simulink library "ob_alb_fov"  (Simulink 6.2)
undefined symbols (not defined in the file or in its folder): albedo_onboard_wrapper, zenith2ref
libraries: components_lib x5, simulink x1, sensor_emulation_lib x1
settings Model: Creator=rsni02  LastModifiedBy=rsni02  ExtModeAutoUpdateStatusClock=off

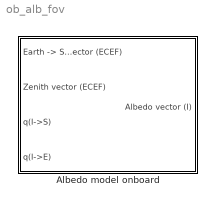
== system ob_alb_fov ==
  Albedo model onboard : Subsystem  mask{sun_flux=1366.9, matrix=FOV cosine dep. reflectivity table, enable=off}
      mask prompts: sun_flux "Sun flux (mean: 1366.9)"; matrix "Choose used reflectivity data:"; enable "Use reflectivity matrix (blackbox)"
      mask init:
      | if matrix == 1
      |     mrm = load('fov_albedo_matrix.mat');
      |     mrm = mrm.mrm;  
      | elseif matrix == 2
      |     mrm = load('fov_meaned_albedo_matrix.mat');
      |     mrm = mrm.mrm;
      | elseif matrix == 3
      |     mrm = load('fov_albedo_polynomial_matrix.mat');
      |     mrm = mrm.mrm;
      | elseif matrix == 4
      |     mrm = ones(180,288).*0.30;
      | end
      mask StyleString: edit,popup(FOV cosine dep. reflectivity table|FOV meaned reflectivity table|Polynomial fit to latitude meaned reflectivity|Constant reflectivity of 30%),checkbox

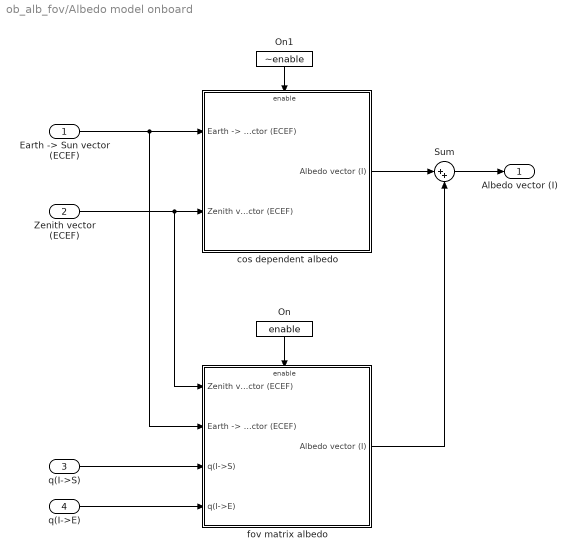
== system ob_alb_fov/Albedo model onboard ==
  "Earth -> Sun vector (ECEF)" : Inport  Port=1  LatchInput=off
  Zenith vector (ECEF) : Inport  Port=2  LatchInput=off
  q(I->S) : Inport  Port=3  LatchInput=off
  q(I->E) : Inport  Port=4  LatchInput=off
  On : Constant  Orientation=down  Value=enable
  On1 : Constant  Orientation=down  Value=~enable
  Sum : Sum  Inputs=|++
  cos dependent albedo : Subsystem
  fov matrix albedo : Subsystem
  Albedo vector (I) : Outport
  wires:
  On1/1 -> cos dependent albedo/Enable
  fov matrix albedo/1(Albedo vector (I)) -> Sum/2
  cos dependent albedo/1(Albedo vector (I)) -> Sum/1
  On/1 -> fov matrix albedo/Enable
  Zenith vector (ECEF)/1 -> fov matrix albedo/1(Zenith vector (ECEF)), cos dependent albedo/2(Zenith vector (ECEF))
  "Earth -> Sun vector (ECEF)"/1 -> fov matrix albedo/2("Earth -> Sun vector (ECEF)"), cos dependent albedo/1("Earth -> Sun vector (ECEF)")
  q(I->E)/1 -> fov matrix albedo/4(q(I->E))
  q(I->S)/1 -> fov matrix albedo/3(q(I->S))
  Sum/1 -> Albedo vector (I)/1

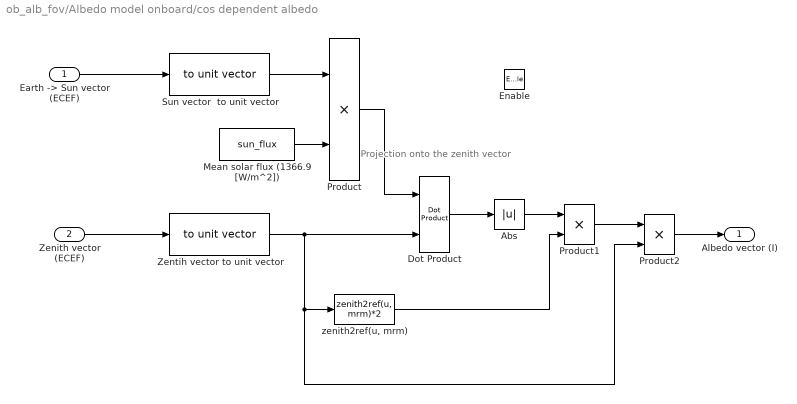
== system ob_alb_fov/Albedo model onboard/cos dependent albedo ==
  note: Projection onto
      | the zenith vector
  "Earth -> Sun vector (ECEF)" : Inport  Port=1  LatchInput=off
  Zenith vector (ECEF) : Inport  Port=2  LatchInput=off
  Enable : EnablePort  StatesWhenEnabling=reset
  Abs : Abs
  Dot Product : simulink/Math Operations/Dot Product  InputSameDT=on  OutDataType=sfix(16)  OutScaling=2^-10  DoSatur=off
  Mean solar flux (1366.9 [W/m^2]) : Constant  Value=sun_flux
  Product : Product  RndMeth=Zero
  Product1 : Product  RndMeth=Zero
  Product2 : Product  RndMeth=Zero
  Sun vector  to unit vector : components_lib/Math utilities/Vector operations/to unit vector
  Zentih vector to unit vector : components_lib/Math utilities/Vector operations/to unit vector
  "zenith2ref(u, mrm)" : MATLABFcn  MATLABFcn=zenith2ref(u, mrm)*2
  Albedo vector (I) : Outport
  wires:
  Product2/1 -> Albedo vector (I)/1
  Product1/1 -> Product2/1
  Abs/1 -> Product1/1
  Dot Product/1 -> Abs/1
  Sun vector  to unit vector/1 -> Product/1
  Mean solar flux (1366.9 [W/m^2])/1 -> Product/2
  Product/1 -> Dot Product/1
  "zenith2ref(u, mrm)"/1 -> Product1/2
  Zentih vector to unit vector/1 -> Product2/2, "zenith2ref(u, mrm)"/1, Dot Product/2
  "Earth -> Sun vector (ECEF)"/1 -> Sun vector  to unit vector/1
  Zenith vector (ECEF)/1 -> Zentih vector to unit vector/1

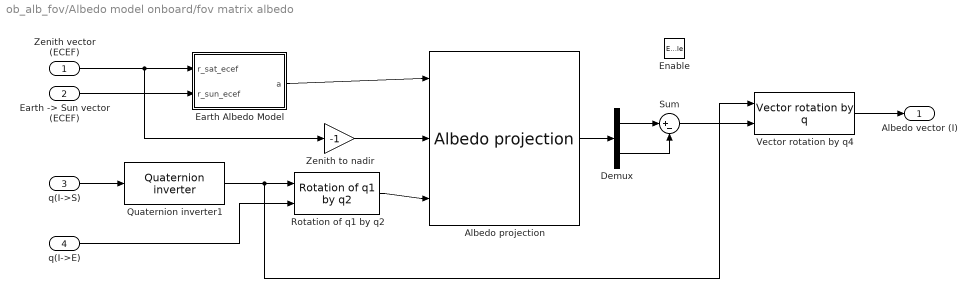
== system ob_alb_fov/Albedo model onboard/fov matrix albedo ==
  Zenith vector (ECEF) : Inport  Port=1  LatchInput=off
  "Earth -> Sun vector (ECEF)" : Inport  Port=2  LatchInput=off
  q(I->S) : Inport  Port=3  LatchInput=off
  q(I->E) : Inport  Port=4  LatchInput=off
  Enable : EnablePort  StatesWhenEnabling=reset
  Albedo projection : sensor_emulation_lib/Sensor Emulation/Sun sensors/sun sensor model/Albedo projection
  Demux : Demux  Outputs=2
  Earth Albedo Model : Subsystem  TreatAsAtomicUnit=on  mask(Earth Albedo Model){eprdata=load('lib/space_environment_emulation/albedo/toolbox/epr_data/2003/ga030101-031231'), redfac=10, Ts=1, enable=on}
      mask prompts: eprdata "Reflectivity Data (EPR Struct):"; redfac "Reduction factor:"; Ts "Sample Time (-1 for inherited):"
      mask help: Calculate Earth Albedo using static data from the EP/TOMS spacecraft.
      mask init:
      | global sy;
      | global sx;
      | sy = round(180/redfac);
      | sx = round(288/redfac);
      mask Help:
      | <b>Input</b><br>
      | Sat: Vector to satellite in ECEF [m]<br>
      | Sun: Vector to the Sun in ECEF [m]<p>
      | <b>Parameters</b><br>
      | Reflectivity Data (EPR Struct): TOMS Reflectivity data [E.U].<br>
      | Reduction factor: Reduce data resolution by this factor.<br>
      | Sample Time (-1 for inherited): Sample Time [s]. The block cannot inherit continuous sample time.<br>
      | Enable: Enable or disable albedo calculation<p>
      | <b>Output</b><br>
      | Albedo: Fraction of solar irradiance received on the satellite. The incoming solar irradiance is 1366.5 W/m^2<p>
      mask CallbackString: |||enable = strcmp(get_param(gcb,'enable'),'on');
      mask Display:
      | image(imread('private/albedoicon.png'));
      | port_label('output', 1, 'Albedo');
      | port_label('input', 1, 'Sat');
      | port_label('input', 2, 'Sun');
  Quaternion inverter1 : components_lib/Math utilities/Quaternion operations/Quaternion inverter
  Rotation of q1 by q2 : components_lib/Math utilities/Quaternion operations/Rotation of q1 by q2
  Sum : Sum  Inputs=|+-
  Vector rotation by q4 : components_lib/Math utilities/Quaternion operations/Vector rotation by q
  "Zenith to nadir " : Gain  Gain=-1
  Albedo vector (I) : Outport
  wires:
  "Earth -> Sun vector (ECEF)"/1 -> Earth Albedo Model/2(r_sun_ecef)
  Zenith vector (ECEF)/1 -> "Zenith to nadir "/1, Earth Albedo Model/1(r_sat_ecef)
  Vector rotation by q4/1 -> Albedo vector (I)/1
  q(I->E)/1 -> Rotation of q1 by q2/2
  q(I->S)/1 -> Quaternion inverter1/1
  Earth Albedo Model/1(a) -> Albedo projection/1
  "Zenith to nadir "/1 -> Albedo projection/2
  Quaternion inverter1/1 -> Rotation of q1 by q2/1, Vector rotation by q4/1
  Rotation of q1 by q2/1 -> Albedo projection/3
  Albedo projection/1 -> Demux/1
  Demux/1 -> Sum/1
  Demux/2 -> Sum/2
  Sum/1 -> Vector rotation by q4/2

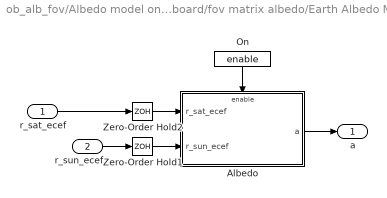
== system ob_alb_fov/Albedo model onboard/fov matrix albedo/Earth Albedo Model ==
  r_sat_ecef : Inport  Port=1  SampleTime=Ts  LatchInput=off
  r_sun_ecef : Inport  Port=2  SampleTime=Ts  LatchInput=off
  Albedo : Subsystem
  On : Constant  Orientation=down  Value=enable
  Zero-Order Hold1 : ZeroOrderHold  SampleTime=Ts
  Zero-Order Hold2 : ZeroOrderHold  SampleTime=Ts
  a : Outport
  wires:
  Zero-Order Hold1/1 -> Albedo/2(r_sun_ecef)
  Zero-Order Hold2/1 -> Albedo/1(r_sat_ecef)
  r_sun_ecef/1 -> Zero-Order Hold1/1
  Albedo/1(a) -> a/1
  r_sat_ecef/1 -> Zero-Order Hold2/1
  On/1 -> Albedo/Enable

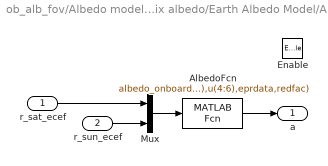
== system ob_alb_fov/Albedo model onboard/fov matrix albedo/Earth Albedo Model/Albedo ==
  r_sat_ecef : Inport  Port=1  PortDimensions=3  LatchInput=off
  r_sun_ecef : Inport  Port=2  PortDimensions=3  LatchInput=off
  Enable : EnablePort  StatesWhenEnabling=reset
  AlbedoFcn : MATLABFcn  MATLABFcn=albedo_onboard_wrapper(u(1:3),u(4:6),eprdata,redfac)  OutputDimensions=floor([180 288]./redfac)  OutputSignalType=real  Output1D=off
  Mux : Mux  Inputs=2
  a : Outport  OutputWhenDisabled=reset  InitialOutput=0
  wires:
  Mux/1 -> AlbedoFcn/1
  r_sat_ecef/1 -> Mux/1
  AlbedoFcn/1 -> a/1
  r_sun_ecef/1 -> Mux/2
